simulink library "INT_EISGov_TrqLosEst"  (R2016b)
settings: Solver=VariableStepAuto  StartTime=0.0  StopTime=10.0  RelTol=1e-3
settings Model: Creator=xuxingpei  LastModifiedBy=xuxingpei

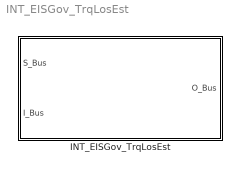
== system INT_EISGov_TrqLosEst ==
  INT_EISGov_TrqLosEst : Subsystem

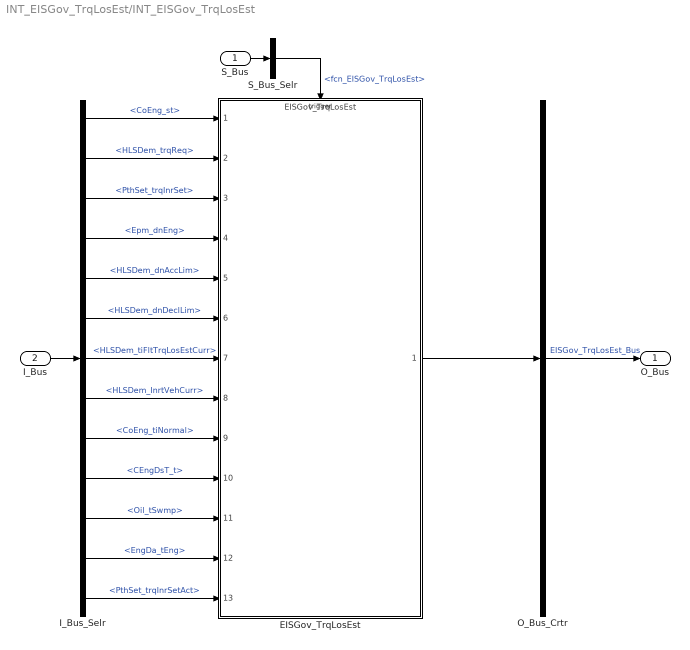
== system INT_EISGov_TrqLosEst/INT_EISGov_TrqLosEst ==
  S_Bus : Inport
  I_Bus : Inport  Port=2
  EISGov_TrqLosEst : ModelReference  ModelNameDialog=EISGov_TrqLosEst  SimulationMode=Normal  ModelReferenceVersion=1.93  TriggerPortName=function  TriggerPortTriggerType=function-call  TriggerPortStatesWhenEnabling=held
  I_Bus_Selr : BusSelector  OutputSignals=CoEng_st,HLSDem_trqReq,PthSet_trqInrSet,Epm_dnEng,HLSDem_dnAccLim,HLSDem_dnDeclLim,HLSDem_tiFltTrqLosEstCurr,HLSDem_InrtVehCurr,CoEng_tiNormal,CEngDsT_t,Oil_tSwmp,EngDa_tEng,PthSet_trqInrSetAct
  O_Bus_Crtr : BusCreator  Inputs=1
  S_Bus_Selr : BusSelector  OutputSignals=fcn_EISGov_TrqLosEst
  O_Bus : Outport
  wires:
  S_Bus_Selr/1 -> EISGov_TrqLosEst/Trigger  "<fcn_EISGov_TrqLosEst>"
  S_Bus/1 -> S_Bus_Selr/1
  I_Bus/1 -> I_Bus_Selr/1
  I_Bus_Selr/1 -> EISGov_TrqLosEst/1  "<CoEng_st>"
  I_Bus_Selr/2 -> EISGov_TrqLosEst/2  "<HLSDem_trqReq>"
  I_Bus_Selr/3 -> EISGov_TrqLosEst/3  "<PthSet_trqInrSet>"
  I_Bus_Selr/4 -> EISGov_TrqLosEst/4  "<Epm_dnEng>"
  I_Bus_Selr/5 -> EISGov_TrqLosEst/5  "<HLSDem_dnAccLim>"
  I_Bus_Selr/6 -> EISGov_TrqLosEst/6  "<HLSDem_dnDeclLim>"
  I_Bus_Selr/7 -> EISGov_TrqLosEst/7  "<HLSDem_tiFltTrqLosEstCurr>"
  I_Bus_Selr/8 -> EISGov_TrqLosEst/8  "<HLSDem_InrtVehCurr>"
  I_Bus_Selr/9 -> EISGov_TrqLosEst/9  "<CoEng_tiNormal>"
  I_Bus_Selr/10 -> EISGov_TrqLosEst/10  "<CEngDsT_t>"
  I_Bus_Selr/11 -> EISGov_TrqLosEst/11  "<Oil_tSwmp>"
  I_Bus_Selr/12 -> EISGov_TrqLosEst/12  "<EngDa_tEng>"
  I_Bus_Selr/13 -> EISGov_TrqLosEst/13  "<PthSet_trqInrSetAct>"
  O_Bus_Crtr/1 -> O_Bus/1  "EISGov_TrqLosEst_Bus"
  EISGov_TrqLosEst/1 -> O_Bus_Crtr/1
